simulink model "model_one_upgrade3"  (R2025b)
settings: Solver=VariableStepAuto  StartTime=0.0  StopTime=1000000  RelTol=1e-3
undefined symbols (not defined in the file or in its folder): battery_builder_rtmsupport, gcbh
libraries: nesl_utility x14, fl_lib x8, dspstat3 x6, BatteryEstimators x3, BatteryProtection x3, batt_lib x2, Batteries_Pack_lib x2, BatteriesLASTNOTLEAST_lib x2, BatterySoeEstimators x2, autolibshared x1, mqttlib x1, BatteryBalancing x1
(part 3 of 3)

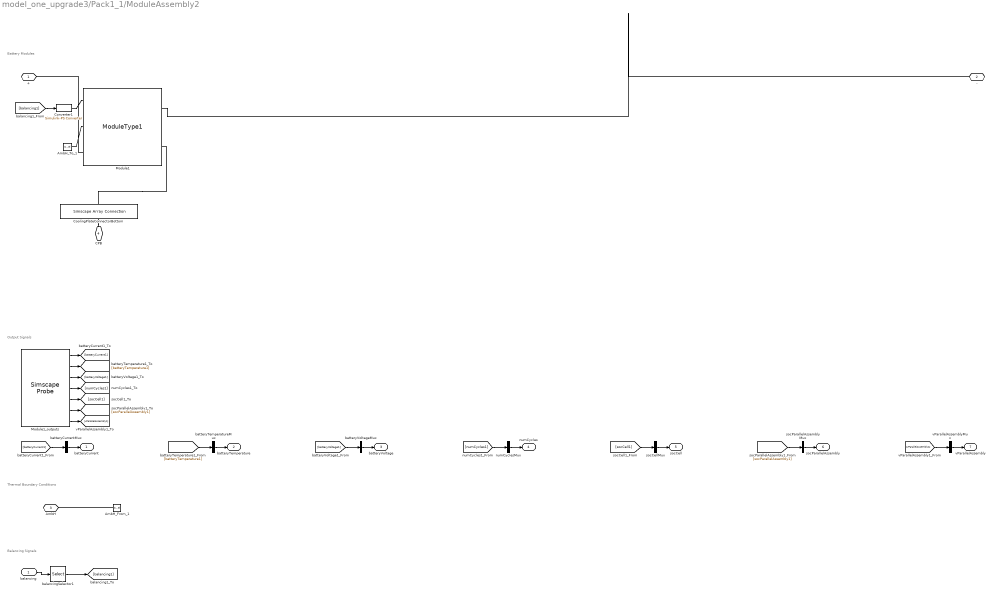
== system model_one_upgrade3/Pack1_1/ModuleAssembly2 ==
  note: Battery Modules
  note: Output Signals
  note: Thermal Boundary Conditions
  note: Balancing Signals
  balancing : Inport  PortDimensions=2
  AmbH_From_1 : ConnectionLabel  Label=ambH_1
  AmbH_To_1 : ConnectionLabel  Label=ambH_1
  Converter1 : nesl_utility/Simulink-PS Converter  PhysicalDomain=network_engine_domain  SubClassName=ps_input  LeftPortType=input  RightPortType=output  PseudoPeriodic=off  Frequencies=[]  NoiseDistribution=none  NoiseParameters=[]  Unit=1  AffineConversion=off  FilteringAndDerivatives=provide  SimscapeFilterOrder=1  InputFilterTimeConstant=0.001  UdotUserProvided=0
  CoolingPlateConnectorBottom : SimscapeArrayConnection  Domain=foundation.thermal.thermal  Mode=Sized Elements
  Module1 : BatteriesLASTNOTLEAST_lib/Modules/ModuleType1  BatteryCapacityCell=ModuleAssembly2.Module1.BatteryCapacityCell A*hr  ExtrapolationMethodCell=simscape.enum.extrapolation.linear  SOCBreakpointsCell=ModuleAssembly2.Module1.SOCBreakpointsCell  TemperatureBreakpointsCell=ModuleAssembly2.Module1.TemperatureBreakpointsCell degC  OpenCircuitVoltageThermalCell=ModuleAssembly2.Module1.OpenCircuitVoltageThermalCell V  VoltageRangeCell=ModuleAssembly2.Module1.VoltageRangeCell V  ResistanceSOCBreakpointsCell=ModuleAssembly2.Module1.ResistanceSOCBreakpointsCell  ResistanceTemperatureBreakpointsCell=ModuleAssembly2.Module1.ResistanceTemperatureBreakpointsCell degC  R0ThermalCell=ModuleAssembly2.Module1.R0ThermalCell Ohm  BatteryThermalMassCell=ModuleAssembly2.Module1.BatteryThermalMassCell J/K  CoolantResistance=ModuleAssembly2.Module1.CoolantResistance K/W  AmbientResistance=ModuleAssembly2.Module1.AmbientResistance K/W  InterCellThermalResistance=ModuleAssembly2.Module1.InterCellThermalResistance K/W  InterParallelAssemblyThermalResistance=ModuleAssembly2.Module1.InterParallelAssemblyThermalResistance K/W  CellBalancingClosedResistance=ModuleAssembly2.Module1.CellBalancingClosedResistance Ohm  CellBalancingOpenConductance=ModuleAssembly2.Module1.CellBalancingOpenConductance 1/Ohm  CellBalancingThreshold=ModuleAssembly2.Module1.CellBalancingThreshold  CellBalancingResistance=ModuleAssembly2.Module1.CellBalancingResistance Ohm  P=2  S=2  NumInterCellThermalConnections=2  NumInterParallelAssemblyThermalConnections=4  InterParallelAssemblyConnectionsMapping=[1, 1, 1, 1; 2, 2, 2, 2]  InterParallelAssemblyCellConnectionsMapping=[1, 1, 2, 2; 1, 2, 1, 2]  InterCellConnectionsMapping=[1, 1; 2, 2]  socCell_specify=off  socCell_priority=High  socCell=repmat(1, 4, 1)  socCell_nominal_specify=off  socCell_nominal_value=1  socCell_nominal_unit=1  batteryVoltage_specify=off  batteryVoltage_priority=None  batteryVoltage=repmat(0, 4, 1) V  batteryVoltage_nominal_specify=off  batteryVoltage_nominal_value=1  batteryVoltage_nominal_unit=V  batteryCurrent_specify=off  batteryCurrent_priority=None  batteryCurrent=repmat(0, 4, 1) A  batteryCurrent_nominal_specify=off  batteryCurrent_nominal_value=1  batteryCurrent_nominal_unit=A  numCycles_specify=off  numCycles_priority=High  numCycles=repmat(0, 4, 1)  numCycles_nominal_specify=off  numCycles_nominal_value=1  numCycles_nominal_unit=1  batteryTemperature_specify=off  batteryTemperature_priority=High  batteryTemperature=repmat(298.15, 4, 1) K  batteryTemperature_nominal_specify=off  batteryTemperature_nominal_value=1  batteryTemperature_nominal_unit=K  vParallelAssembly_specify=off  vParallelAssembly_priority=None  vParallelAssembly=repmat(0, 2, 1) V  vParallelAssembly_nominal_specify=off  vParallelAssembly_nominal_value=1  vParallelAssembly_nominal_unit=V  socParallelAssembly_specify=off  socParallelAssembly_priority=None  socParallelAssembly=repmat(1, 2, 1)  socParallelAssembly_nominal_specify=off  socParallelAssembly_nominal_value=1  socParallelAssembly_nominal_unit=1
      settings: InternalSimscapePortConfiguration="{\"Bottom\":[{\"id\":\"n\",\"label\":\"-\",\"type\":\"foundation.electrical.electrical\"},{\"id\":\"BottomExtClnt\",\"label\":\"CPB\",\"type\":\"foundation.thermal.thermal\"}],\"Left\":[{\"id\":\"enableCellBalancing\",\"label\":\"CB\",\"type\":\"input\"},{\"id\":\"AmbH\",\"label\":\"AmbH\",\"type\":\"foundation.thermal.thermal\"}],\"Right\":[],\"Top\":[{\"id\":\"p\",\"label\":\"+\",\"type\":\"foundation.electrical.electrical\"}]}"
  Module1_outputs : SimscapeProbe  BoundBlock=1081  Variables="{\"batteryCurrent\":{\"Probing\":\"ON\"},\"batteryTemperature\":{\"Probing\":\"ON\"},\"batteryVoltage\":{\"Probing\":\"ON\"},\"numCycles\":{\"Probing\":\"ON\"},\"socCell\":{\"Probing\":\"ON\"},\"socParallelAssembly\":{\"Probing\":\"ON\"},\"vParallelAssembly\":{\"Probing\":\"ON\"}}"
  balancingSelector1 : Selector  InputPortWidth=2  IndexOptions=Index vector (dialog)  Indices="[1  2]"  OutputSizes=1
  batteryCurrentMux : Mux  Inputs=1
  batteryTemperatureMux : Mux  Inputs=1
  batteryVoltageMux : Mux  Inputs=1
  numCyclesMux : Mux  Inputs=1
  socCellMux : Mux  Inputs=1
  socParallelAssemblyMux : Mux  Inputs=1
  vParallelAssemblyMux : Mux  Inputs=1
  + : PMIOPort  Side=Left
  - : PMIOPort  Port=2  Side=Right
  AmbH : PMIOPort  Port=3  Side=Right  ConnectionType=Connection: foundation.thermal.thermal
  CPB : PMIOPort  Port=4  Side=Right  ConnectionType=Connection: foundation.thermal.thermal
  batteryCurrent : Outport
  batteryTemperature : Outport  Port=2
  batteryVoltage : Outport  Port=3
  numCycles : Outport  Port=4
  socCell : Outport  Port=5
  socParallelAssembly : Outport  Port=6
  vParallelAssembly : Outport  Port=7
  wires:
  Module1_outputs/1 -> [batteryCurrent1]
  batteryCurrentMux/1 -> batteryCurrent/1
  [batteryCurrent1] -> batteryCurrentMux/1
  Module1_outputs/2 -> [batteryTemperature1]
  batteryTemperatureMux/1 -> batteryTemperature/1
  [batteryTemperature1] -> batteryTemperatureMux/1
  Module1_outputs/3 -> [batteryVoltage1]
  batteryVoltageMux/1 -> batteryVoltage/1
  [batteryVoltage1] -> batteryVoltageMux/1
  Module1_outputs/4 -> [numCycles1]
  numCyclesMux/1 -> numCycles/1
  [numCycles1] -> numCyclesMux/1
  Module1_outputs/5 -> [socCell1]
  socCellMux/1 -> socCell/1
  [socCell1] -> socCellMux/1
  Module1_outputs/6 -> [socParallelAssembly1]
  socParallelAssemblyMux/1 -> socParallelAssembly/1
  [socParallelAssembly1] -> socParallelAssemblyMux/1
  Module1_outputs/7 -> [vParallelAssembly1]
  vParallelAssemblyMux/1 -> vParallelAssembly/1
  [vParallelAssembly1] -> vParallelAssemblyMux/1
  [balancing1] -> Converter1/1
  balancing/1 -> balancingSelector1/1
  balancingSelector1/1 -> [balancing1]
  connections:
  Module1/LConn3 -- +/RConn1
  Module1/RConn1 -- -/RConn1
  Converter1/RConn1 -- Module1/LConn1
  AmbH_To_1/LConn1 -- Module1/LConn2
  AmbH_From_1/LConn1 -- AmbH/RConn1
  CoolingPlateConnectorBottom/LConn1 -- Module1/RConn2
  CoolingPlateConnectorBottom/RConn1 -- CPB/RConn1

== matlab function model_one_upgrade3/Calculate The Electrical Power ==
  data: v input; Current output; a input; V_batt_act input
function Current = calc_current(v, a, V_batt_act)
    % --- الثوابت الخاصة بالسيارة (تقدر تعدلها حسب وزن عربيتك) ---
    m = 500;       % كتلة السيارة (kg)
    g = 9.81;       % الجاذبية الأرضية (m/s^2)
    rho = 1.225;    % كثافة الهواء (kg/m^3)
    Cd = 0.3;       % معامل مقاومة الهواء
    A = 2.0;        % المساحة الأمامية للسيارة (m^2)
    Cr = 0.015;     % معامل مقاومة التدحرج
    eff = 0.85;     % كفاءة الموتور والمنظومة

    % --- 1. حساب القوى الديناميكية ---
    F_acc = m * a;
    F_drag = 0.5 * rho * Cd * A * (v^2);
    F_roll = m * g * Cr;
    
    F_total = F_acc + F_drag + F_roll;
    
    % --- 2. حساب القدرة الميكانيكية والكهربائية ---
    P_mech = F_total * v;
    
    if P_mech >= 0
        P_elec = P_mech / eff; 
    else
        P_elec = P_mech * eff; 
    end
    
    % --- 3. حساب التيار (أمبير) بناءً على فولت التست الحقيقي ---
    % حماية منطقية: لو الفولت قليل جداً أو صفر لتجنب القسمة على صفر
    if V_batt_act > 1
        Current = P_elec / V_batt_act;
    else
        Current = 0;
    end
    
    % حماية عند التوقف
    if v <= 0.01 && a <= 0
        Current = 0;
    end
end

== matlab function model_one_upgrade3/MQTT_Pblisher/MATLAB Function ==
  data: current input; jsonOut output uint8 size=[1, 1000]; temp input; voltage input; soc input; cycles input; total_soc input; SOH input
function jsonOut = fcn(current, temp, voltage, soc, cycles, total_soc, SOH)
    % 1. تأمين تحويل المصفوفات الأساسية لفيكتورات أفقية
    c = current(:)';
    t = temp(:)';
    v = voltage(:)';
    s = soc(:)';
    cy = cycles(:)';
    ts = total_soc(:)';
    
    % 2. تأمين متغير الـ SOH كقيمة مفردة أفقية
    sh = SOH(:)';

    % 3. بناء الـ JSON وتنسيق الـ SOH في آخر الملف
    rawJson = sprintf(['{\n', ...
                       '  "current": [%.2f, %.2f, %.2f, %.2f, %.2f, %.2f, %.2f, %.2f],\n', ...
                       '  "temp": [%.2f, %.2f, %.2f, %.2f, %.2f, %.2f, %.2f, %.2f],\n', ...
                       '  "voltage": [%.2f, %.2f, %.2f, %.2f, %.2f, %.2f, %.2f, %.2f],\n', ...
                       '  "soc": [%.2f, %.2f, %.2f, %.2f, %.2f, %.2f, %.2f, %.2f],\n', ...
                       '  "cycles": [%.2f, %.2f, %.2f, %.2f, %.2f, %.2f, %.2f, %.2f],\n', ...
                       '  "total_soc": [%.2f],\n', ...
                       '  "SOH": %.2f\n', ...
                       '}'], ...
                       c(1), c(2), c(3), c(4), c(5), c(6), c(7), c(8), ...
                       t(1), t(2), t(3), t(4), t(5), t(6), t(7), t(8), ...
                       v(1), v(2), v(3), v(4), v(5), v(6), v(7), v(8), ...
                       s(1), s(2), s(3), s(4), s(5), s(6), s(7), s(8), ...
                       cy(1), cy(2), cy(3), cy(4), cy(5), cy(6), cy(7), cy(8), ...
                       ts(1), sh(1));
                  
    % 4. حجز مصفوفة الأصفار (Null Bytes) لسلامة الـ JSON Parser
    % حجم 1000 بايت كافي جداً ومريح الآن بعد تقليل المتغيرات
    jsonOut = zeros(1, 1000, 'uint8');
    
    % 5. نقل النص إلى مصفوفة الـ uint8 مع حماية الأبعاد
    len = length(rawJson);
    if len > 1000
        len = 1000;
    end
    jsonOut(1:len) = uint8(rawJson(1:len));
end
